simulink library "MAVLink_library"  (Simulink 3.00)
undefined symbols (not defined in the file): diag______, ERR, I32, I64, INFO, Large, Long, MAV, MAV_AUTOPILOT_GENERIC, WARN, yenum
libraries: mathlib x37, logiclib x35, stringlib x30, analoglib x8, mavlinklib x8, paramlib x4, execlib x3, genlib x2, MAVLink_library x1, timelib x1
settings Model: MaskType=REX sequence  MaskIconFrame=on  MaskIconOpaque=on  MaskIconRotate=none  MaskIconUnits=autoscale

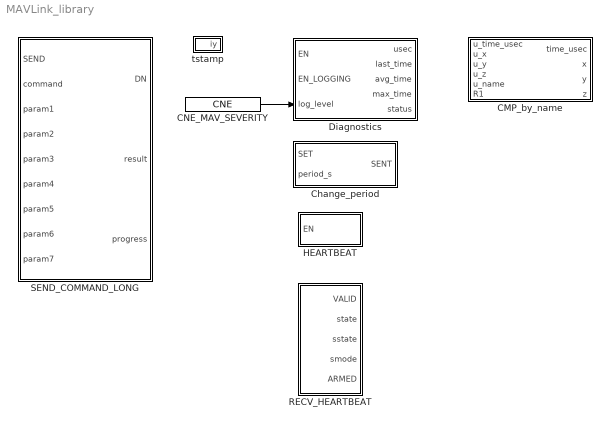
== system MAVLink_library ==
  CMP_by_name : Subsystem  mask(REX sequence){name=diag______}
  CNE_MAV_SEVERITY : mathlib/CNE  yenum=6: Info  pupstr=3: Error|4: Warning|6: Info|7: Verbose
  Change_period : Subsystem  mask(REX sequence){TgtSysID=254, TgtCompID=173}
  Diagnostics : Subsystem  mask(REX sequence){SrcSystemID=254, SrcComponentID=173}
  HEARTBEAT : Subsystem  mask(REX sequence){TgtSysID=-1, MAV_TYPE=0}
      mask prompts: TgtSysID "Target SysID"; MAV_TYPE "MAV_TYPE 0:GENERIC 18:ON_BOARD 31:CHARGING_STATION"
  RECV_HEARTBEAT : Subsystem  mask(REX sequence){SysID=1}
      mask prompts: SysID "System ID of the MAVLink device"
  SEND_COMMAND_LONG : Subsystem  mask(REX sequence){TgtSysID=, TgtCompID=, Timeout=1}
      mask prompts: TgtSysID "Target system ID"; TgtCompID "Target component ID"; Timeout "Timeout in secods when command will be repeated"
  tstamp : Subsystem
      mask Type: REX sequence
  wires:
  CNE_MAV_SEVERITY/1 -> Diagnostics/3(log_level)

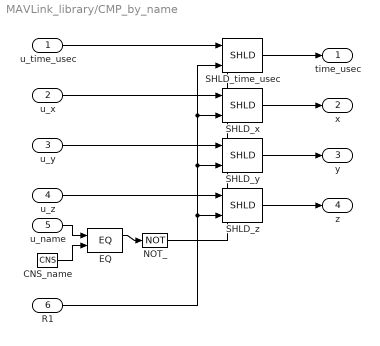
== system MAVLink_library/CMP_by_name ==
  u_time_usec : Inport  Port=1  OutDataTypeStr=Inherit: auto
  u_x : Inport  Port=2  OutDataTypeStr=Inherit: auto
  u_y : Inport  Port=3  OutDataTypeStr=Inherit: auto
  u_z : Inport  Port=4  OutDataTypeStr=Inherit: auto
  u_name : Inport  Port=5  OutDataTypeStr=Inherit: auto
  R1 : Inport  Port=6  OutDataTypeStr=Inherit: auto
  CNS_name : stringlib/CNS  scv=name  nmax=0
  EQ : logiclib/EQ
  NOT_ : logiclib/NOT
  SHLD_time_usec : analoglib/SHLD  y0=0  mode=2: Hold last value
  SHLD_x : analoglib/SHLD  y0=0  mode=2: Hold last value
  SHLD_y : analoglib/SHLD  y0=0  mode=2: Hold last value
  SHLD_z : analoglib/SHLD  y0=0  mode=2: Hold last value
  time_usec : Outport  Port=1  OutDataTypeStr=Inherit: auto
  x : Outport  Port=2  OutDataTypeStr=Inherit: auto
  y : Outport  Port=3  OutDataTypeStr=Inherit: auto
  z : Outport  Port=4  OutDataTypeStr=Inherit: auto
  wires:
  CNS_name/1 -> EQ/2
  EQ/1 -> NOT_/1
  NOT_/1 -> SHLD_time_usec/2, SHLD_x/2, SHLD_y/2, SHLD_z/2
  R1/1 -> SHLD_z/3, SHLD_y/3, SHLD_time_usec/3, SHLD_x/3
  SHLD_time_usec/1 -> time_usec/1
  SHLD_x/1 -> x/1
  SHLD_y/1 -> y/1
  SHLD_z/1 -> z/1
  u_name/1 -> EQ/1
  u_time_usec/1 -> SHLD_time_usec/1
  u_x/1 -> SHLD_x/1
  u_y/1 -> SHLD_y/1
  u_z/1 -> SHLD_z/1

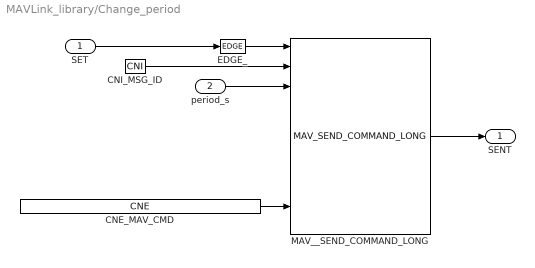
== system MAVLink_library/Change_period ==
  SET : Inport  Port=1  OutDataTypeStr=Inherit: auto
  period_s : Inport  Port=2  OutDataTypeStr=Inherit: auto
  CNE_MAV_CMD : mathlib/CNE  yenum=511: MAV_CMD_SET_MESSAGE_INTERVAL  pupstr=511: MAV_CMD_SET_MESSAGE_INTERVAL
  CNI_MSG_ID : mathlib/CNI  icn=0  vtype=4: Long (I32)
  EDGE_ : logiclib/EDGE  iedge=1: Rising edge
  MAV__SEND_COMMAND_LONG : mavlinklib/MAV_SEND_COMMAND_LONG  TgtSysID=TgtSysID  TgtCompID=TgtCompID
  SENT : Outport  Port=1  OutDataTypeStr=Inherit: auto
  wires:
  CNE_MAV_CMD/1 -> MAV__SEND_COMMAND_LONG/9
  CNI_MSG_ID/1 -> MAV__SEND_COMMAND_LONG/2
  EDGE_/1 -> MAV__SEND_COMMAND_LONG/1
  MAV__SEND_COMMAND_LONG/1 -> SENT/1
  SET/1 -> EDGE_/1
  period_s/1 -> MAV__SEND_COMMAND_LONG/3

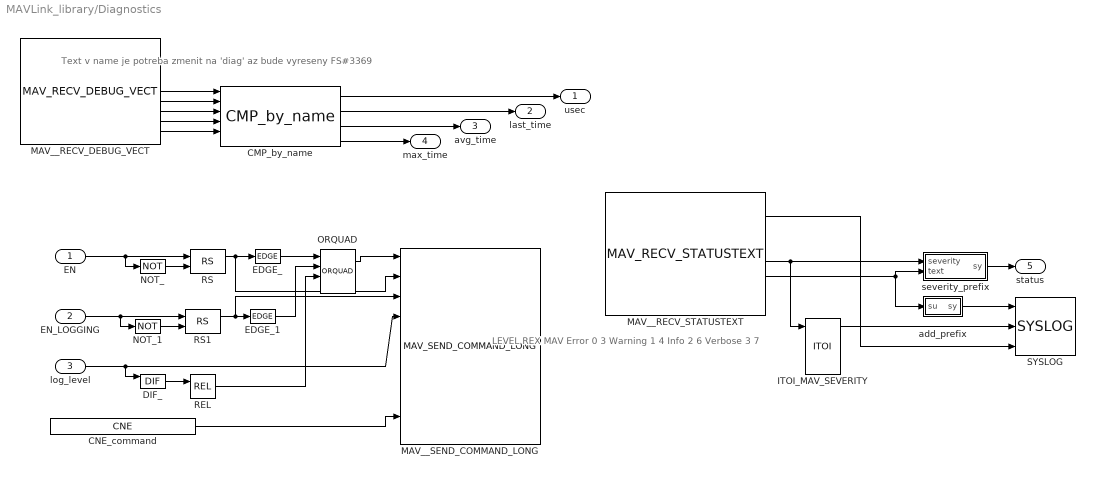
== system MAVLink_library/Diagnostics ==
  note: LEVEL    REX MAV
      | Error        0      3
      | Warning  1      4
      | Info         2      6
      | Verbose   3      7
  note: Text v name je potreba zmenit na 'diag' az bude vyreseny FS#3369
  EN : Inport  Port=1  OutDataTypeStr=Inherit: auto
  EN_LOGGING : Inport  Port=2  OutDataTypeStr=Inherit: auto
  log_level : Inport  Port=3  OutDataTypeStr=Inherit: auto
  CMP_by_name : MAVLink_library/CMP_by_name  name=diag______
  CNE_command : mathlib/CNE  yenum=31013: MAV_CMD_USER_4  pupstr=31010: MAV_CMD_USER_1|31011: MAV_CMD_USER_2|31012: MAV_CMD_USER_3|31013: MAV_CMD_USER_4
  DIF_ : mathlib/DIF  ISSF=off
  EDGE_ : logiclib/EDGE  iedge=3: Both edges
  EDGE_1 : logiclib/EDGE  iedge=3: Both edges
  ITOI_MAV_SEVERITY : logiclib/ITOI  BINF=off  fktab=[0 0 0 0 1 2 2 3 3 3 3 3 3 3 3 3]
  MAV__RECV_DEBUG_VECT : mavlinklib/MAV_RECV_DEBUG_VECT  SrcSystemID=254  SrcComponentID=173  TgtSystemID=-1  TgtComponentID=-1  TimeoutMS=0
  MAV__RECV_STATUSTEXT : mavlinklib/MAV_RECV_STATUSTEXT  SrcSystemID=SrcSystemID  SrcComponentID=SrcComponentID  TgtSystemID=-1  TgtComponentID=-1  TimeoutMS=0
  MAV__SEND_COMMAND_LONG : mavlinklib/MAV_SEND_COMMAND_LONG  TgtSysID=SrcSystemID  TgtCompID=SrcComponentID  SrcSysID=-1  SrcCompID=-1
  NOT_ : logiclib/NOT
  NOT_1 : logiclib/NOT
  ORQUAD : logiclib/ORQUAD  nl=0
  REL : mathlib/REL  irel=2: inequality (!=)
  RS : logiclib/RS
  RS1 : logiclib/RS
  SYSLOG : execlib/SYSLOG
  add_prefix : Subsystem  mask(REX sequence){prefix=[MAV]:}
  severity_prefix : Subsystem
      mask Type: REX sequence
  usec : Outport  Port=1  OutDataTypeStr=Inherit: auto
  last_time : Outport  Port=2  OutDataTypeStr=Inherit: auto
  avg_time : Outport  Port=3  OutDataTypeStr=Inherit: auto
  max_time : Outport  Port=4  OutDataTypeStr=Inherit: auto
  status : Outport  Port=5  OutDataTypeStr=Inherit: auto
  wires:
  CMP_by_name/1 -> usec/1
  CMP_by_name/2 -> last_time/1
  CMP_by_name/3 -> avg_time/1
  CMP_by_name/4 -> max_time/1
  CNE_command/1 -> MAV__SEND_COMMAND_LONG/9
  DIF_/1 -> REL/1
  EDGE_/1 -> ORQUAD/1
  EDGE_1/1 -> ORQUAD/2
  EN/1 -> NOT_/1, RS/1
  EN_LOGGING/1 -> NOT_1/1, RS1/1
  ITOI_MAV_SEVERITY/1 -> SYSLOG/2
  MAV__RECV_DEBUG_VECT/5 -> CMP_by_name/1
  MAV__RECV_DEBUG_VECT/6 -> CMP_by_name/2
  MAV__RECV_DEBUG_VECT/7 -> CMP_by_name/3
  MAV__RECV_DEBUG_VECT/8 -> CMP_by_name/4
  MAV__RECV_DEBUG_VECT/9 -> CMP_by_name/5
  MAV__RECV_STATUSTEXT/2 -> SYSLOG/3
  MAV__RECV_STATUSTEXT/5 -> ITOI_MAV_SEVERITY/1, severity_prefix/1(severity)
  MAV__RECV_STATUSTEXT/6 -> add_prefix/1(su), severity_prefix/2(text)
  NOT_/1 -> RS/2
  NOT_1/1 -> RS1/2
  ORQUAD/1 -> MAV__SEND_COMMAND_LONG/1
  REL/1 -> ORQUAD/3
  RS/1 -> EDGE_/1, MAV__SEND_COMMAND_LONG/2
  RS1/1 -> EDGE_1/1, MAV__SEND_COMMAND_LONG/3
  add_prefix/1(sy) -> SYSLOG/1
  log_level/1 -> DIF_/1, MAV__SEND_COMMAND_LONG/4
  severity_prefix/1(sy) -> status/1

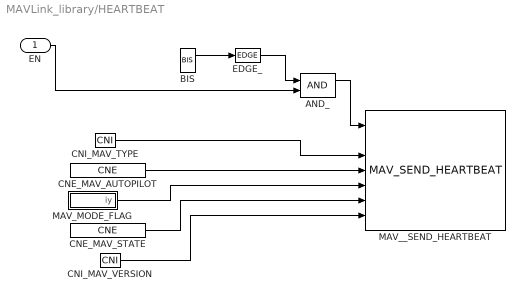
== system MAVLink_library/HEARTBEAT ==
  EN : Inport  Port=1  OutDataTypeStr=Inherit: auto
  AND_ : logiclib/AND
  BIS : genlib/BIS  Y0=off  t1=0.5  t2=1  t3=0  t4=4  t5=5  t6=6  t7=7  t8=8  RPT=on
  CNE_MAV_AUTOPILOT : mathlib/CNE  yenum=0:MAV_AUTOPILOT_GENERIC  pupstr=0:MAV_AUTOPILOT_GENERIC |8: MAV_AUTOPILOT_INVALID
  CNE_MAV_STATE : mathlib/CNE  yenum=4: MAV_STATE_ACTIVE  pupstr=4: MAV_STATE_ACTIVE
  CNI_MAV_TYPE : mathlib/CNI  icn=MAV_TYPE  vtype=4: Long (I32)
  CNI_MAV_VERSION : mathlib/CNI  icn=3  vtype=4: Long (I32)
  EDGE_ : logiclib/EDGE  iedge=1: Rising edge
  MAV_MODE_FLAG : Subsystem
      mask Type: REX sequence
  MAV__SEND_HEARTBEAT : mavlinklib/MAV_SEND_HEARTBEAT  TgtSysID=TgtSysID  TgtCompID=-1  SrcSysID=-1  SrcCompID=-1
  wires:
  AND_/1 -> MAV__SEND_HEARTBEAT/1
  BIS/1 -> EDGE_/1
  CNE_MAV_AUTOPILOT/1 -> MAV__SEND_HEARTBEAT/4
  CNE_MAV_STATE/1 -> MAV__SEND_HEARTBEAT/6
  CNI_MAV_TYPE/1 -> MAV__SEND_HEARTBEAT/3
  CNI_MAV_VERSION/1 -> MAV__SEND_HEARTBEAT/7
  EDGE_/1 -> AND_/1
  EN/1 -> AND_/2
  MAV_MODE_FLAG/1(iy) -> MAV__SEND_HEARTBEAT/5

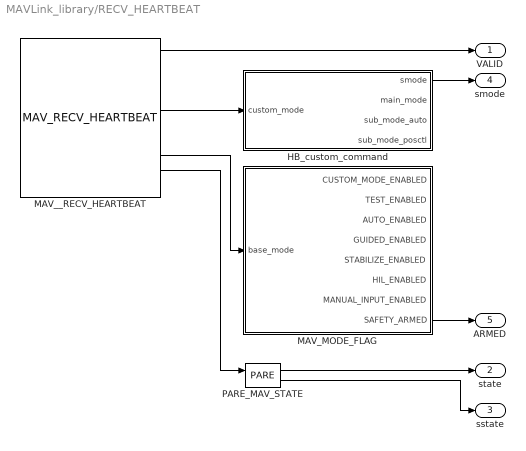
== system MAVLink_library/RECV_HEARTBEAT ==
  HB_custom_command : Subsystem
      mask Type: REX sequence
  MAV_MODE_FLAG : Subsystem
      mask Type: REX sequence
  MAV__RECV_HEARTBEAT : mavlinklib/MAV_RECV_HEARTBEAT  SrcSystemID=SysID  SrcComponentID=1  TgtSystemID=-1  TgtComponentID=-1  TimeoutMS=2000
  PARE_MAV_STATE : paramlib/PARE  ipar=1: BOOT  pupstr=0: UNINIT|1: BOOT|2: CALIBRATING|3: STANDBY|4: ACTIVE|5: CRITICAL|6: EMERGENCY|7: POWEROFF|8: FLIGHT_TERMINATION  NUM=off  LIST=off  SATF=off
  VALID : Outport  Port=1  OutDataTypeStr=Inherit: auto
  state : Outport  Port=2  OutDataTypeStr=Inherit: auto
  sstate : Outport  Port=3  OutDataTypeStr=Inherit: auto
  smode : Outport  Port=4  OutDataTypeStr=Inherit: auto
  ARMED : Outport  Port=5  OutDataTypeStr=Inherit: auto
  wires:
  HB_custom_command/1(smode) -> smode/1
  MAV_MODE_FLAG/8(SAFETY_ARMED) -> ARMED/1
  MAV__RECV_HEARTBEAT/1 -> VALID/1
  MAV__RECV_HEARTBEAT/5 -> HB_custom_command/1(custom_mode)
  MAV__RECV_HEARTBEAT/8 -> MAV_MODE_FLAG/1(base_mode)
  MAV__RECV_HEARTBEAT/9 -> PARE_MAV_STATE/1
  PARE_MAV_STATE/1 -> state/1
  PARE_MAV_STATE/2 -> sstate/1

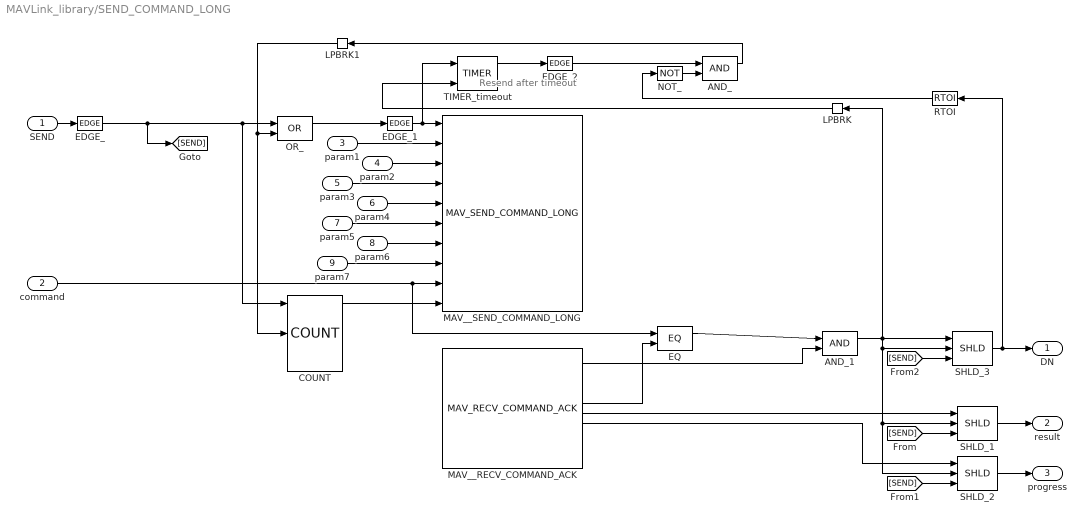
== system MAVLink_library/SEND_COMMAND_LONG ==
  note: Resend after timeout
  SEND : Inport  Port=1  OutDataTypeStr=Inherit: auto
  command : Inport  Port=2  OutDataTypeStr=Inherit: auto
  param1 : Inport  Port=3  OutDataTypeStr=Inherit: auto
  param2 : Inport  Port=4  OutDataTypeStr=Inherit: auto
  param3 : Inport  Port=5  OutDataTypeStr=Inherit: auto
  param4 : Inport  Port=6  OutDataTypeStr=Inherit: auto
  param5 : Inport  Port=7  OutDataTypeStr=Inherit: auto
  param6 : Inport  Port=8  OutDataTypeStr=Inherit: auto
  param7 : Inport  Port=9  OutDataTypeStr=Inherit: auto
  AND_ : logiclib/AND
  AND_1 : logiclib/AND
  COUNT : logiclib/COUNT
  EDGE_ : logiclib/EDGE  iedge=1: Rising edge
  EDGE_1 : logiclib/EDGE  iedge=1: Rising edge
  EDGE_2 : logiclib/EDGE  iedge=2: Falling edge
  EQ : logiclib/EQ
  LPBRK : execlib/LPBRK  Orientation=left
  LPBRK1 : execlib/LPBRK  Orientation=left
  MAV__RECV_COMMAND_ACK : mavlinklib/MAV_RECV_COMMAND_ACK  SrcSystemID=TgtSysID  SrcComponentID=TgtCompID  TgtSystemID=-1  TgtComponentID=-1  TimeoutMS=0
  MAV__SEND_COMMAND_LONG : mavlinklib/MAV_SEND_COMMAND_LONG  TgtSysID=TgtSysID  TgtCompID=TgtCompID  SrcSysID=-1  SrcCompID=-1
  NOT_ : logiclib/NOT
  OR_ : logiclib/OR
  RTOI : mathlib/RTOI  Orientation=left  vtype=4: Long (I32)  SAT=on
  SHLD_1 : analoglib/SHLD  y0=0  mode=1: Triggered sampling
  SHLD_2 : analoglib/SHLD  y0=0  mode=1: Triggered sampling
  SHLD_3 : analoglib/SHLD  y0=0  mode=1: Triggered sampling
  TIMER_timeout : logiclib/TIMER  mode=1: Pulse generator  pt=Timeout
  DN : Outport  Port=1  OutDataTypeStr=Inherit: auto
  result : Outport  Port=2  OutDataTypeStr=Inherit: auto
  progress : Outport  Port=3  OutDataTypeStr=Inherit: auto
  wires:
  AND_/1 -> LPBRK1/1
  AND_1/1 -> SHLD_1/2, SHLD_2/2, SHLD_3/2, LPBRK/1, SHLD_3/1
  COUNT/1 -> MAV__SEND_COMMAND_LONG/10
  EDGE_/1 -> COUNT/1, OR_/1, [SEND]
  EDGE_1/1 -> MAV__SEND_COMMAND_LONG/1, TIMER_timeout/1
  EDGE_2/1 -> AND_/1
  EQ/1 -> AND_1/1
  [SEND] -> SHLD_1/3
  [SEND] -> SHLD_2/3
  [SEND] -> SHLD_3/3
  LPBRK/1 -> TIMER_timeout/3
  LPBRK1/1 -> COUNT/4, OR_/2
  MAV__RECV_COMMAND_ACK/1 -> AND_1/2
  MAV__RECV_COMMAND_ACK/5 -> EQ/2
  MAV__RECV_COMMAND_ACK/6 -> SHLD_1/1
  MAV__RECV_COMMAND_ACK/7 -> SHLD_2/1
  NOT_/1 -> AND_/2
  OR_/1 -> EDGE_1/1
  RTOI/1 -> NOT_/1
  SEND/1 -> EDGE_/1
  SHLD_1/1 -> result/1
  SHLD_2/1 -> progress/1
  SHLD_3/1 -> DN/1, RTOI/1
  TIMER_timeout/1 -> EDGE_2/1
  command/1 -> EQ/1, MAV__SEND_COMMAND_LONG/9
  param1/1 -> MAV__SEND_COMMAND_LONG/2
  param2/1 -> MAV__SEND_COMMAND_LONG/3
  param3/1 -> MAV__SEND_COMMAND_LONG/4
  param4/1 -> MAV__SEND_COMMAND_LONG/5
  param5/1 -> MAV__SEND_COMMAND_LONG/6
  param6/1 -> MAV__SEND_COMMAND_LONG/7
  param7/1 -> MAV__SEND_COMMAND_LONG/8

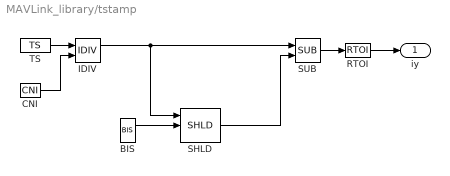
== system MAVLink_library/tstamp ==
  BIS : genlib/BIS  Y0=off  t1=0.1  t2=1  t3=0  t4=4  t5=5  t6=6  t7=7  t8=8  RPT=off
  CNI : mathlib/CNI  icn=1000000  vtype=4: Long (I32)
  IDIV : mathlib/IDIV  vtype=10: Large (I64)  nerr=1
  RTOI : mathlib/RTOI  vtype=4: Long (I32)  SAT=on
  SHLD : analoglib/SHLD  y0=0  mode=1: Triggered sampling
  SUB : mathlib/SUB
  TS : timelib/TS  source=1
  iy : Outport  Port=1  OutDataTypeStr=Inherit: auto
  wires:
  BIS/1 -> SHLD/2
  CNI/1 -> IDIV/2
  IDIV/1 -> SHLD/1, SUB/1
  RTOI/1 -> iy/1
  SHLD/1 -> SUB/2
  SUB/1 -> RTOI/1
  TS/1 -> IDIV/1

== system MAVLink_library/Diagnostics/add_prefix ==
  su : Inport  Port=1  OutDataTypeStr=Inherit: auto
  CNS : stringlib/CNS  scv=prefix  nmax=0
  CONCAT : stringlib/CONCAT  ptrn=%1%2  nmax=0
  sy : Outport  Port=1  OutDataTypeStr=Inherit: auto
  wires:
  CNS/1 -> CONCAT/1
  CONCAT/1 -> sy/1
  su/1 -> CONCAT/2

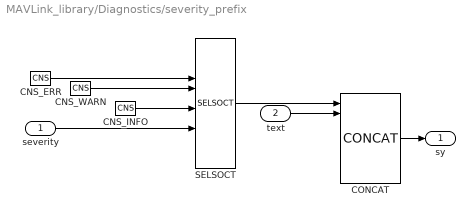
== system MAVLink_library/Diagnostics/severity_prefix ==
  severity : Inport  Port=1  OutDataTypeStr=Inherit: auto
  text : Inport  Port=2  OutDataTypeStr=Inherit: auto
  CNS_ERR : stringlib/CNS  scv=[ERR]:  nmax=0
  CNS_INFO : stringlib/CNS  scv=[INFO]:  nmax=0
  CNS_WARN : stringlib/CNS  scv=[WARN]:  nmax=0
  CONCAT : stringlib/CONCAT  ptrn=%1%2  nmax=0
  SELSOCT : stringlib/SELSOCT  BINF=off  nmax=0
  sy : Outport  Port=1  OutDataTypeStr=Inherit: auto
  wires:
  CNS_ERR/1 -> SELSOCT/4
  CNS_INFO/1 -> SELSOCT/7
  CNS_WARN/1 -> SELSOCT/5
  CONCAT/1 -> sy/1
  SELSOCT/1 -> CONCAT/1
  severity/1 -> SELSOCT/9
  text/1 -> CONCAT/2

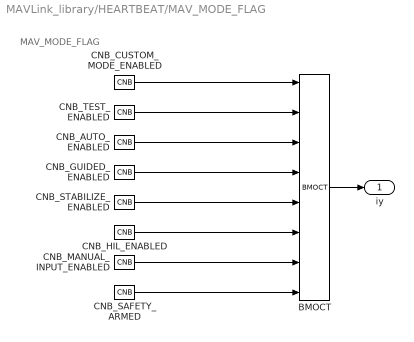
== system MAVLink_library/HEARTBEAT/MAV_MODE_FLAG ==
  note: MAV_MODE_FLAG
  BMOCT : logiclib/BMOCT  shift=0  vtype=4: Long (I32)
  CNB_AUTO_ENABLED : mathlib/CNB  YCN=off
  CNB_CUSTOM_MODE_ENABLED : mathlib/CNB  YCN=off
  CNB_GUIDED_ENABLED : mathlib/CNB  YCN=off
  CNB_HIL_ENABLED : mathlib/CNB  YCN=off
  CNB_MANUAL_INPUT_ENABLED : mathlib/CNB  YCN=on
  CNB_SAFETY_ARMED : mathlib/CNB  YCN=on
  CNB_STABILIZE_ENABLED : mathlib/CNB  YCN=off
  CNB_TEST_ENABLED : mathlib/CNB  YCN=off
  iy : Outport  Port=1  OutDataTypeStr=Inherit: auto
  wires:
  BMOCT/1 -> iy/1
  CNB_AUTO_ENABLED/1 -> BMOCT/3
  CNB_CUSTOM_MODE_ENABLED/1 -> BMOCT/1
  CNB_GUIDED_ENABLED/1 -> BMOCT/4
  CNB_HIL_ENABLED/1 -> BMOCT/6
  CNB_MANUAL_INPUT_ENABLED/1 -> BMOCT/7
  CNB_SAFETY_ARMED/1 -> BMOCT/8
  CNB_STABILIZE_ENABLED/1 -> BMOCT/5
  CNB_TEST_ENABLED/1 -> BMOCT/2

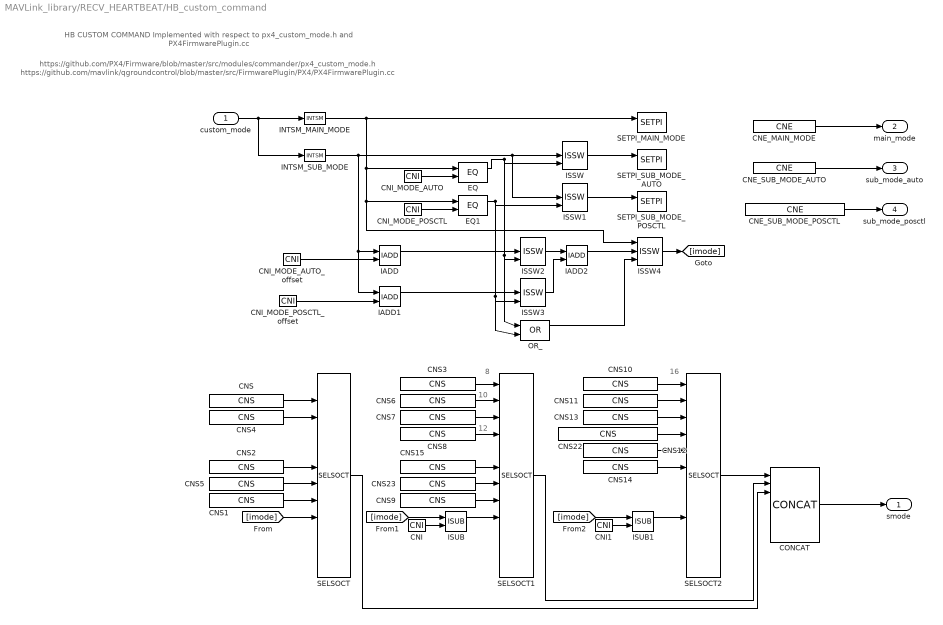
== system MAVLink_library/RECV_HEARTBEAT/HB_custom_command ==
  note: 8
  note: 16
  note: 10
  note: 12
  note: https://github.com/PX4/Firmware/blob/master/src/modules/commander/px4_custom_mode.h
      |
      | https://github.com/mavlink/qgroundcontrol/blob/master/src/FirmwarePlugin/PX4/PX4FirmwarePlugin.cc
  note: HB CUSTOM COMMAND
      | Implemented with respect to px4_custom_mode.h and PX4FirmwarePlugin.cc
  custom_mode : Inport  Port=1  OutDataTypeStr=Inherit: auto
  CNE_MAIN_MODE : mathlib/CNE  yenum=0: NOT SET  pupstr=0: NOT SET|1: MANUAL|2: ALTCTL|3: POSCTL|4: AUTO|5: ACRO|6: OFFBOARD|7: STABILIZED|8: RATTITUDE|9: SIMPLE
  CNE_SUB_MODE_AUTO : mathlib/CNE  yenum=0:  pupstr=0:|1: READY|2: TAKEOFF|3: LOITER|4: MISSION|5: RTL|6: LAND|7: RTGS|8: FOLLOW_TARGET|9: PRECLAND
  CNE_SUB_MODE_POSCTL : mathlib/CNE  yenum=0: POSCTL  pupstr=0: POSCTL| 1: ORBIT
  CNI : mathlib/CNI  icn=8  vtype=4: Long (I32)
  CNI1 : mathlib/CNI  icn=16  vtype=4: Long (I32)
  CNI_MODE_AUTO : mathlib/CNI  icn=4  vtype=4: Long (I32)
  CNI_MODE_AUTO_offset : mathlib/CNI  icn=12  vtype=4: Long (I32)
  CNI_MODE_POSCTL : mathlib/CNI  icn=3  vtype=4: Long (I32)
  CNI_MODE_POSCTL_offset : mathlib/CNI  icn=10  vtype=4: Long (I32)
  CNS : stringlib/CNS  scv=Manual  nmax=0
  CNS1 : stringlib/CNS  scv=Stabilized  nmax=0
  CNS10 : stringlib/CNS  scv=Mission  nmax=0
  CNS11 : stringlib/CNS  scv=Return  nmax=0
  CNS12 : stringlib/CNS  scv=Follow Me  nmax=0
  CNS13 : stringlib/CNS  scv=Land  nmax=0
  CNS14 : stringlib/CNS  scv=Precision Land  nmax=0
  CNS15 : stringlib/CNS  scv=Ready  nmax=0
  CNS2 : stringlib/CNS  scv=Acro  nmax=0
  CNS22 : stringlib/CNS  scv=Return to Groundstation  nmax=0
  CNS23 : stringlib/CNS  scv=Takeoff  nmax=0
  CNS3 : stringlib/CNS  scv=Rattitude  nmax=0
  CNS4 : stringlib/CNS  scv=Altitude  nmax=0
  CNS5 : stringlib/CNS  scv=Offboard  nmax=0
  CNS6 : stringlib/CNS  scv=Simple  nmax=0
  CNS7 : stringlib/CNS  scv=Position  nmax=0
  CNS8 : stringlib/CNS  scv=Orbit  nmax=0
  CNS9 : stringlib/CNS  scv=Hold  nmax=0
  CONCAT : stringlib/CONCAT  ptrn=%1%2%3%4  nmax=0
  EQ : logiclib/EQ
  EQ1 : logiclib/EQ
  IADD : mathlib/IADD  vtype=4: Long (I32)  SAT=off
  IADD1 : mathlib/IADD  vtype=4: Long (I32)  SAT=off
  IADD2 : mathlib/IADD  vtype=4: Long (I32)  SAT=off
  INTSM_MAIN_MODE : logiclib/INTSM  shift=16  mask=255  vtype=10: Large (I64)
  INTSM_SUB_MODE : logiclib/INTSM  shift=24  mask=255  vtype=10: Large (I64)
  ISSW{,1..4} (5 alike) : logiclib/ISSW
  ISUB : mathlib/ISUB  vtype=4: Long (I32)  SAT=off
  ISUB1 : mathlib/ISUB  vtype=4: Long (I32)  SAT=off
  OR_ : logiclib/OR
  SELSOCT : stringlib/SELSOCT  BINF=off  nmax=0
  SELSOCT1 : stringlib/SELSOCT  BINF=off  nmax=0
  SELSOCT2 : stringlib/SELSOCT  BINF=off  nmax=0
  SETPI_MAIN_MODE : paramlib/SETPI  sc=.CNE_MAIN_MODE:yenum  SETF=off
  SETPI_SUB_MODE_AUTO : paramlib/SETPI  sc=.CNE_SUB_MODE_AUTO:yenum  SETF=off
  SETPI_SUB_MODE_POSCTL : paramlib/SETPI  sc=.CNE_SUB_MODE_POSCTL:yenum  SETF=off
  smode : Outport  Port=1  OutDataTypeStr=Inherit: auto
  main_mode : Outport  Port=2  OutDataTypeStr=Inherit: auto
  sub_mode_auto : Outport  Port=3  OutDataTypeStr=Inherit: auto
  sub_mode_posctl : Outport  Port=4  OutDataTypeStr=Inherit: auto
  wires:
  CNE_MAIN_MODE/1 -> main_mode/1
  CNE_SUB_MODE_AUTO/1 -> sub_mode_auto/1
  CNE_SUB_MODE_POSCTL/1 -> sub_mode_posctl/1
  CNI/1 -> ISUB/2
  CNI1/1 -> ISUB1/2
  CNI_MODE_AUTO/1 -> EQ/2
  CNI_MODE_AUTO_offset/1 -> IADD/2
  CNI_MODE_POSCTL/1 -> EQ1/2
  CNI_MODE_POSCTL_offset/1 -> IADD1/2
  CNS/1 -> SELSOCT/2
  CNS1/1 -> SELSOCT/8
  CNS10/1 -> SELSOCT2/1
  CNS11/1 -> SELSOCT2/2
  CNS12/1 -> SELSOCT2/5
  CNS13/1 -> SELSOCT2/3
  CNS14/1 -> SELSOCT2/6
  CNS15/1 -> SELSOCT1/6
  CNS2/1 -> SELSOCT/6
  CNS22/1 -> SELSOCT2/4
  CNS23/1 -> SELSOCT1/7
  CNS3/1 -> SELSOCT1/1
  CNS4/1 -> SELSOCT/3
  CNS5/1 -> SELSOCT/7
  CNS6/1 -> SELSOCT1/2
  CNS7/1 -> SELSOCT1/3
  CNS8/1 -> SELSOCT1/4
  CNS9/1 -> SELSOCT1/8
  CONCAT/1 -> smode/1
  EQ/1 -> ISSW/3, ISSW2/3, OR_/1
  EQ1/1 -> ISSW1/3, ISSW3/3, OR_/2
  [imode] -> SELSOCT/9
  [imode] -> ISUB/1
  [imode] -> ISUB1/1
  IADD/1 -> ISSW2/2
  IADD1/1 -> ISSW3/2
  IADD2/1 -> ISSW4/2
  INTSM_MAIN_MODE/1 -> SETPI_MAIN_MODE/1, EQ/1, EQ1/1, ISSW4/1
  INTSM_SUB_MODE/1 -> ISSW/2, ISSW1/2, IADD/1, IADD1/1
  ISSW/1 -> SETPI_SUB_MODE_AUTO/1
  ISSW1/1 -> SETPI_SUB_MODE_POSCTL/1
  ISSW2/1 -> IADD2/1
  ISSW3/1 -> IADD2/2
  ISSW4/1 -> [imode]
  ISUB/1 -> SELSOCT1/9
  ISUB1/1 -> SELSOCT2/9
  OR_/1 -> ISSW4/3
  SELSOCT/1 -> CONCAT/3
  SELSOCT1/1 -> CONCAT/2
  SELSOCT2/1 -> CONCAT/1
  custom_mode/1 -> INTSM_MAIN_MODE/1, INTSM_SUB_MODE/1

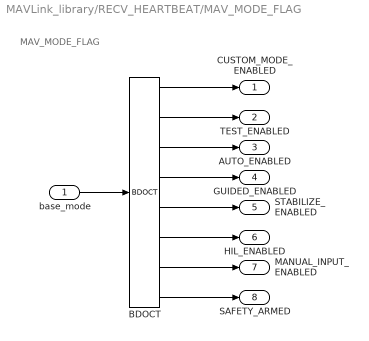
== system MAVLink_library/RECV_HEARTBEAT/MAV_MODE_FLAG ==
  note: MAV_MODE_FLAG
  base_mode : Inport  Port=1  OutDataTypeStr=Inherit: auto
  BDOCT : logiclib/BDOCT  shift=0  vtype=4: Long (I32)
  CUSTOM_MODE_ENABLED : Outport  Port=1  OutDataTypeStr=Inherit: auto
  TEST_ENABLED : Outport  Port=2  OutDataTypeStr=Inherit: auto
  AUTO_ENABLED : Outport  Port=3  OutDataTypeStr=Inherit: auto
  GUIDED_ENABLED : Outport  Port=4  OutDataTypeStr=Inherit: auto
  STABILIZE_ENABLED : Outport  Port=5  OutDataTypeStr=Inherit: auto
  HIL_ENABLED : Outport  Port=6  OutDataTypeStr=Inherit: auto
  MANUAL_INPUT_ENABLED : Outport  Port=7  OutDataTypeStr=Inherit: auto
  SAFETY_ARMED : Outport  Port=8  OutDataTypeStr=Inherit: auto
  wires:
  BDOCT/1 -> CUSTOM_MODE_ENABLED/1
  BDOCT/2 -> TEST_ENABLED/1
  BDOCT/3 -> AUTO_ENABLED/1
  BDOCT/4 -> GUIDED_ENABLED/1
  BDOCT/5 -> STABILIZE_ENABLED/1
  BDOCT/6 -> HIL_ENABLED/1
  BDOCT/7 -> MANUAL_INPUT_ENABLED/1
  BDOCT/8 -> SAFETY_ARMED/1
  base_mode/1 -> BDOCT/1
